simulink model "LocalPlannerIndexer"  (R2024b)
settings: Solver=VariableStepAuto  StartTime=0.0  StopTime=inf  FixedStep=0.02  RelTol=1e-3
StartFcn:
  | clf
  | rng(1,"twister");
settings Model: Creator=cstabile  LastModifiedBy=apattass
settings DataIOCC: SaveOutput=off  SaveTime=off
settings OptimizationCC: BlockReduction=off  EnhancedBackFolding=on  PassReuseOutputArgsAs=Individual arguments  ZeroExternalMemoryAtStartup=off  ZeroInternalMemoryAtStartup=off  MaxStackSize=64  OptimizeBlockOrder=speed  DifferentSizesBufferReuse=on  OptimizationCustomize=off  EfficientTunableParamExpr=on
settings DebuggingCC: IntegerOverflowMsg=none  ParameterTunabilityLossMsg=error
settings ModelReferenceCC: UpdateModelReferenceTargets=IfOutOfDate
settings SFSimCC: SFSimEcho=off  SimTargetLang=C++
settings RTWCC: Description=Embedded Coder  SystemTargetFile=ert.tlc  TemplateMakefile=ert_default_tmf  Toolchain=Colcon Tools  GPUComputeCapability=3.5
settings CodeAppCC: ForceParamTrailComments=on  IgnoreCustomStorageClasses=off  OperatorAnnotations=on  SimulinkDataObjDesc=on  SFDataObjDesc=on  InsertBlockDesc=on
settings ERTTargetCC: InlinedParameterPlacement=Hierarchical  RootIOFormat=Structure reference  ERTCustomFileTemplate=example_file_process.tlc  DynamicArrayContainerType=coder::array

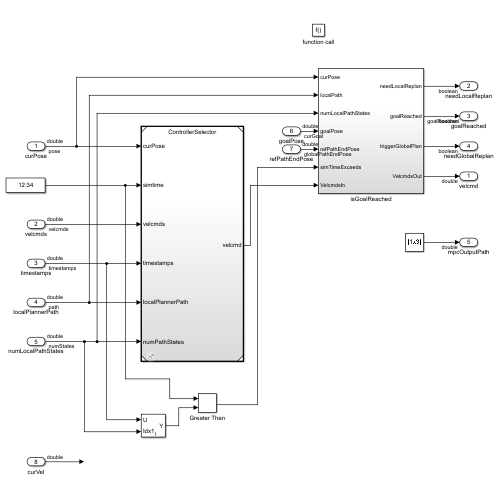
[thumbnail: Simulink's stored preview of the top-level diagram]
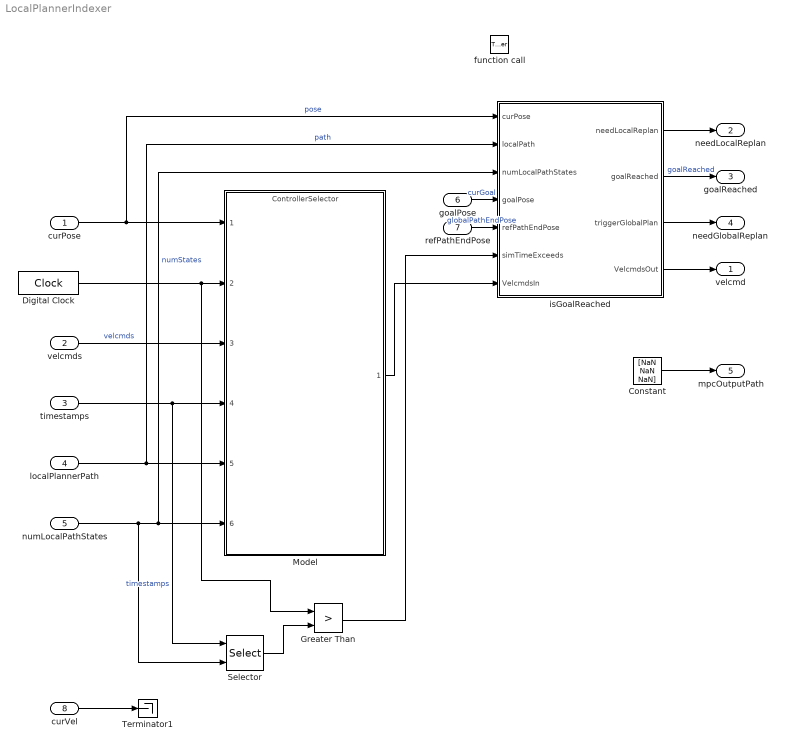
== system LocalPlannerIndexer ==
  curPose : Inport  OutDataTypeStr=double  PortDimensions=[1 3]
  velcmds : Inport  Port=2  OutDataTypeStr=double  PortDimensions=[1000 2]
  timestamps : Inport  Port=3  OutDataTypeStr=double  PortDimensions=[1000 1]
  localPlannerPath : Inport  Port=4  OutDataTypeStr=double  PortDimensions=[1000 3]
  numLocalPathStates : Inport  Port=5  OutDataTypeStr=double  PortDimensions=1
  goalPose : Inport  Port=6  OutDataTypeStr=double  PortDimensions=[1 3]
  refPathEndPose : Inport  Port=7  OutDataTypeStr=double  PortDimensions=[1 3]
  curVel : Inport  Port=8  OutDataTypeStr=double  PortDimensions=[1 2]
  function call : TriggerPort  TriggerType=function-call  VariantControl=(inherit)  SampleTimeType=periodic  SampleTime=[0.02,0]  PortDimensions=1  TriggerSignalSampleTime=[0.02,0]
  Constant : Constant  Value=[NaN NaN NaN]
  Digital Clock : DigitalClock  SampleTime=-1
  Greater Than : RelationalOperator  Operator=>  OutDataTypeStr=boolean  RndMeth=Simplest  InputSameDT=off
  Model : ModelReference  ModelNameDialog=ControllerSelector.slx  SimulationMode=Normal  ModelReferenceVersion=2.7
  Selector : Selector  NumberOfDimensions=2  InputPortWidth=1  IndexOptions=Index vector (port),Select all  Indices=[1 3],1  OutputSizes=1,1
  Terminator1 : Terminator
  isGoalReached : Subsystem
  velcmd : Outport  OutDataTypeStr=double  PortDimensions=[1 2]  InitialOutput=[0 0]
  needLocalReplan : Outport  Port=2  OutDataTypeStr=boolean  PortDimensions=1  OutputWhenDisabled=reset  InitialOutput=0
  goalReached : Outport  Port=3  OutDataTypeStr=boolean  PortDimensions=1
  needGlobalReplan : Outport  Port=4  OutDataTypeStr=boolean  PortDimensions=1  OutputWhenDisabled=reset  InitialOutput=0
  mpcOutputPath : Outport  Port=5  OutDataTypeStr=double  PortDimensions=[1 3]
  wires:
  Digital Clock/1 -> Model/2, Greater Than/1
  velcmds/1 -> Model/3  "velcmds"
  timestamps/1 -> Model/4, Selector/1  "timestamps"
  localPlannerPath/1 -> Model/5, isGoalReached/2(localPath)  "path"
  numLocalPathStates/1 -> Model/6, isGoalReached/3(numLocalPathStates), Selector/2  "numStates"
  Selector/1 -> Greater Than/2
  curPose/1 -> isGoalReached/1(curPose), Model/1  "pose"
  isGoalReached/2(goalReached) -> goalReached/1  "goalReached"
  isGoalReached/1(needLocalReplan) -> needLocalReplan/1
  refPathEndPose/1 -> isGoalReached/5(refPathEndPose)  "globalPathEndPose"
  curVel/1 -> Terminator1/1
  Greater Than/1 -> isGoalReached/6(simTimeExceeds)
  isGoalReached/3(triggerGlobalPlan) -> needGlobalReplan/1
  goalPose/1 -> isGoalReached/4(goalPose)  "curGoal"
  Model/1 -> isGoalReached/7(VelcmdsIn)
  isGoalReached/4(VelcmdsOut) -> velcmd/1
  Constant/1 -> mpcOutputPath/1

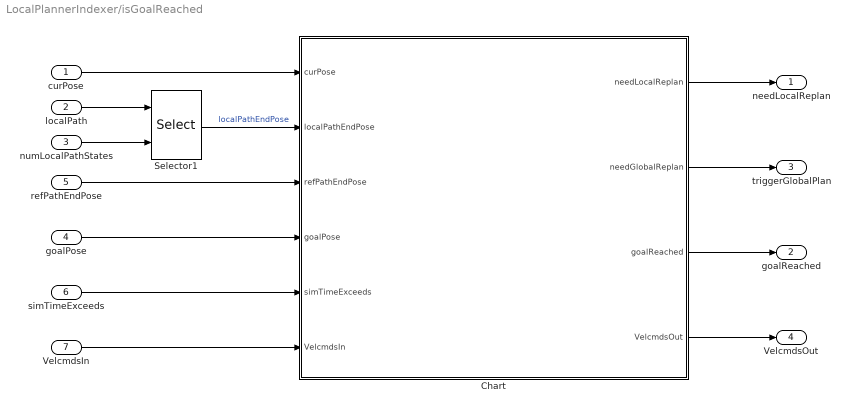
== system LocalPlannerIndexer/isGoalReached ==
  curPose : Inport
  localPath : Inport  Port=2
  numLocalPathStates : Inport  Port=3
  goalPose : Inport  Port=4
  refPathEndPose : Inport  Port=5
  simTimeExceeds : Inport  Port=6
  VelcmdsIn : Inport  Port=7
  Chart : Stateflow chart  TreatAsAtomicUnit=on
      settings: PortSchema="{\"entries\":[{\"content\":{\"sides\":[{\"content\":{\"connectorIds\":[\"In1\",\"In2\",\"In3\",\"In5\",\"In4\",\"In6\"]},\"type\":\"ConnectorPlacement.EquallySpacedRectSide\",\"uuid\":\"dd2a119f-4099-42b7-8b31-d8f3ceb7ac2a\"},{\"content\":{\"connectorIds\":[\"Out1\",\"Out2\",\"Out3\",\"Out4\"],\"side\":\"RIGHT\"},\"type\":\"ConnectorPlacement.EquallySpacedRectSide\",\"uuid\":\"fc746f1f-3a86-4997-a533-2ec7b0a515b4\"},{\"content\":{\"side\":\"TOP\"},\"type\":\"ConnectorPlacement.EquallySpacedRectSide\",\"uuid\":\"464bcae1-c888-4724-83c9-6c7192e3ceb4\"}]},\"type\":\"ConnectorPlacement.EquallySpacedConnector\",\"uuid\":\"b2959aa8-9ba7-43c5-b039-c19b983ed1db\"}],\"packageUris\":[\"http://schema.mathworks.com/mf0/Connector/R2020b\"],\"version\":\"1.0\"}"
  Selector1 : Selector  NumberOfDimensions=2  InputPortWidth=1  IndexOptions=Index vector (port),Select all  Indices=[1 3],1  OutputSizes=1,1
  needLocalReplan : Outport
  goalReached : Outport  Port=2
  triggerGlobalPlan : Outport  Port=3
  VelcmdsOut : Outport  Port=4
  wires:
  Chart/4(VelcmdsOut) -> VelcmdsOut/1
  VelcmdsIn/1 -> Chart/6(VelcmdsIn)
  goalPose/1 -> Chart/5(goalPose)
  simTimeExceeds/1 -> Chart/4(simTimeExceeds)
  Chart/3(goalReached) -> goalReached/1
  Chart/2(needGlobalReplan) -> triggerGlobalPlan/1
  Chart/1(needLocalReplan) -> needLocalReplan/1
  refPathEndPose/1 -> Chart/3(refPathEndPose)
  numLocalPathStates/1 -> Selector1/2
  Selector1/1 -> Chart/2(localPathEndPose)  "localPathEndPose"
  localPath/1 -> Selector1/1
  curPose/1 -> Chart/1(curPose)

== stateflow chart LocalPlannerIndexer/isGoalReached/Chart ==
  (default) -> (junction 6) : {goalTolerance = 4.5;
      | goalReached = false;
      | needGlobalReplan = false;
      | needLocalReplan = false;
      | VelcmdsOut = VelcmdsIn;
      | dist = distBetweenPoses(curPose, goalPose)}
  (junction 6) -> (junction 14) [order 1] : [dist <= goalTolerance]{goalReached = true;}
  (junction 6) -> (junction 16) [order 2] : {dist = distBetweenPoses(curPose, refPathEndPose)}
  (junction 14) -> (junction 18)
  (junction 16) -> (junction 18) [order 1] : [dist <= goalTolerance]{needGlobalReplan = true}
  (junction 16) -> (junction 20) [order 2] : {dist = distBetweenPoses(curPose, localPathEndPose)}
  (junction 18) -> (junction 22) : {VelcmdsOut = [0 0];}
  (junction 20) -> (junction 22) : [dist <= goalTolerance || simTimeExceeds]{needLocalReplan = true}
  data: curpose function_input; nextpose function_input; distOut function_output; curPose input; localPathEndPose input; refPathEndPose input; dist local; goalTolerance local; needLocalReplan output; needGlobalReplan output; goalReached output; simTimeExceeds input; goalPose input; VelcmdsIn input; VelcmdsOut output
  function distOut = distBetweenPoses(curpose, nextpose):
    | function distOut = distBetweenPoses(curpose, nextpose)
    | % distBetweenPoses return the euclidean distance between curpose and nextpose
    |     distOut = vecnorm(curpose(1:2) - nextpose(1:2),2,2);
    | end
